simulink subsystem "SelfDefined_Three_Level_NPC_Converter"  (R2024b)
settings: Solver=VariableStepAuto  StartTime=0.0  StopTime=10.0  RelTol=1e-3
libraries: spsIGBTDiodeLib x12, spsDiodeLib x6, simulink x1
settings Model: Creator=XixiLab  LastModifiedBy=XixiLab

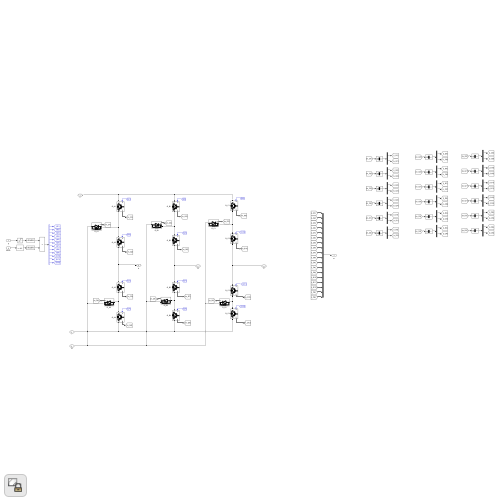
[thumbnail: Simulink's stored preview of the top-level diagram]
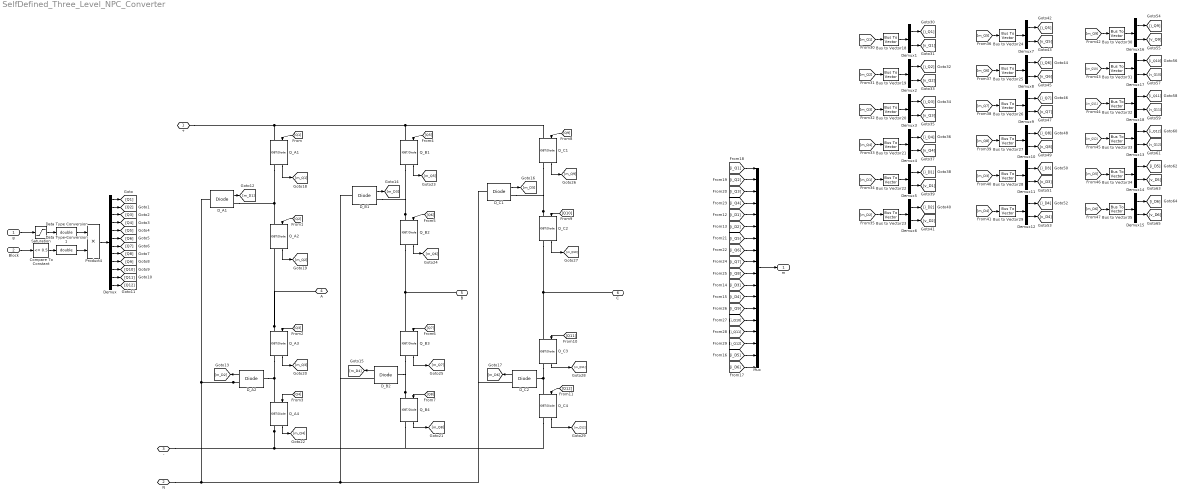
== system SelfDefined_Three_Level_NPC_Converter ==
  g : Inport  PortDimensions=12
  Block : Inport  Port=2  PortDimensions=1
  Bus to Vector{18..35} (18 alike) : BusToVector
  Compare To Constant : simulink/Logic and Bit Operations/Compare To Constant  relop=<=  const=0.5  OutDataTypeStr=boolean
  D_A1 : spsDiodeLib/Diode  Ron=0.001  Lon=0  Vf=0  IC=0  UseSnubber=0  Rs=1e6  Cs=inf  Measurements=on
  D_A2 : spsDiodeLib/Diode  Ron=0.001  Lon=0  Vf=0  IC=0  UseSnubber=0  Rs=1e6  Cs=inf  Measurements=on
  D_B1 : spsDiodeLib/Diode  Ron=0.001  Lon=0  Vf=0  IC=0  UseSnubber=0  Rs=1e6  Cs=inf  Measurements=on
  D_B2 : spsDiodeLib/Diode  Ron=0.001  Lon=0  Vf=0  IC=0  UseSnubber=0  Rs=1e6  Cs=inf  Measurements=on
  D_C1 : spsDiodeLib/Diode  Ron=0.001  Lon=0  Vf=0  IC=0  UseSnubber=0  Rs=1e6  Cs=inf  Measurements=on
  D_C2 : spsDiodeLib/Diode  Ron=0.001  Lon=0  Vf=0  IC=0  UseSnubber=0  Rs=1e6  Cs=inf  Measurements=on
  Data Type Conversion : DataTypeConversion  OutDataTypeStr=double  SaturateOnIntegerOverflow=off  RndMeth=Floor
  Data Type Conversion1 : DataTypeConversion  OutDataTypeStr=double  SaturateOnIntegerOverflow=off  RndMeth=Floor
  Demux : Demux  Outputs=12
  Demux{1..18} (18 alike) : Demux  Outputs=2
  Mux : Mux  Inputs=18
  Product4 : Product
  Q_A{1..4} (4 alike) : spsIGBTDiodeLib/IGBT//Diode  Ron=1e-3  Rs=1e6  Cs=inf  Measurements=on
  Q_B{1..4} (4 alike) : spsIGBTDiodeLib/IGBT//Diode  Ron=1e-3  Rs=1e6  Cs=inf  Measurements=on
  Q_C{1..4} (4 alike) : spsIGBTDiodeLib/IGBT//Diode  Ron=1e-3  Rs=1e6  Cs=inf  Measurements=on
  Saturation : Saturate  UpperLimit=1  LowerLimit=0
  + : PMIOPort  Side=Right
  N : PMIOPort  Port=2  Side=Right
  - : PMIOPort  Port=3  Side=Right
  A : PMIOPort  Port=4  Side=Left
  B : PMIOPort  Port=5  Side=Left
  C : PMIOPort  Port=6  Side=Left
  m : Outport
  wires:
  Demux/10 -> [Q10]
  Data Type Conversion/1 -> Product4/1
  Demux/8 -> [Q8]
  Demux/4 -> [Q4]
  Data Type Conversion1/1 -> Product4/2
  Demux/5 -> [Q5]
  Demux/3 -> [Q3]
  Demux/11 -> [Q11]
  Demux/9 -> [Q9]
  Demux/7 -> [Q7]
  Saturation/1 -> Data Type Conversion/1
  Compare To Constant/1 -> Data Type Conversion1/1
  Demux/6 -> [Q6]
  Product4/1 -> Demux/1
  Demux/12 -> [Q12]
  Demux/2 -> [Q2]
  Demux/1 -> [Q1]
  [Q1] -> Q_A1/1
  [Q2] -> Q_A2/1
  [Q3] -> Q_A3/1
  [Q4] -> Q_A4/1
  [Q6] -> Q_B2/1
  [Q5] -> Q_B1/1
  [Q7] -> Q_B3/1
  [Q8] -> Q_B4/1
  [Q11] -> Q_C3/1
  [Q10] -> Q_C2/1
  [Q12] -> Q_C4/1
  [Q9] -> Q_C1/1
  Block/1 -> Compare To Constant/1
  g/1 -> Saturation/1
  D_A1/1 -> [m_D1]
  D_A2/1 -> [m_D2]
  D_B1/1 -> [m_D3]
  D_B2/1 -> [m_D4]
  D_C1/1 -> [m_D5]
  D_C2/1 -> [m_D6]
  Q_A1/1 -> [m_Q1]
  Q_A2/1 -> [m_Q2]
  Q_A3/1 -> [m_Q3]
  Q_A4/1 -> [m_Q4]
  Q_B1/1 -> [m_Q5]
  Q_B2/1 -> [m_Q6]
  Q_B3/1 -> [m_Q7]
  Q_B4/1 -> [m_Q8]
  Q_C1/1 -> [m_Q9]
  Q_C2/1 -> [m_Q10]
  Q_C3/1 -> [m_Q11]
  Q_C4/1 -> [m_Q12]
  Mux/1 -> m/1
  [i_Q1] -> Mux/1
  [i_Q2] -> Mux/2
  [i_Q3] -> Mux/3
  [i_Q4] -> Mux/4
  [i_D1] -> Mux/5
  [i_D2] -> Mux/6
  [i_Q5] -> Mux/7
  [i_Q6] -> Mux/8
  [i_Q7] -> Mux/9
  [i_Q8] -> Mux/10
  [i_D3] -> Mux/11
  [i_D4] -> Mux/12
  [i_Q9] -> Mux/13
  [i_Q10] -> Mux/14
  [i_Q11] -> Mux/15
  [i_Q12] -> Mux/16
  [i_D5] -> Mux/17
  [i_D6] -> Mux/18
  [m_Q1] -> Bus to Vector18/1
  Bus to Vector18/1 -> Demux1/1
  Demux1/1 -> [i_Q1]
  Demux1/2 -> [v_Q1]
  Demux2/2 -> [v_Q2]
  Bus to Vector19/1 -> Demux2/1
  Demux2/1 -> [i_Q2]
  [m_Q2] -> Bus to Vector19/1
  Demux3/2 -> [v_Q3]
  Bus to Vector20/1 -> Demux3/1
  Demux3/1 -> [i_Q3]
  [m_Q3] -> Bus to Vector20/1
  Demux4/2 -> [v_Q4]
  Bus to Vector21/1 -> Demux4/1
  Demux4/1 -> [i_Q4]
  [m_Q4] -> Bus to Vector21/1
  Demux5/2 -> [v_D1]
  Bus to Vector22/1 -> Demux5/1
  Demux5/1 -> [i_D1]
  [m_D1] -> Bus to Vector22/1
  [m_D2] -> Bus to Vector23/1
  Demux6/1 -> [i_D2]
  Bus to Vector23/1 -> Demux6/1
  Demux6/2 -> [v_D2]
  Demux10/2 -> [v_Q8]
  Bus to Vector27/1 -> Demux10/1
  [m_Q7] -> Bus to Vector26/1
  Demux7/2 -> [v_Q5]
  [m_D3] -> Bus to Vector28/1
  [m_Q6] -> Bus to Vector25/1
  Demux8/2 -> [v_Q6]
  Demux8/1 -> [i_Q6]
  Bus to Vector24/1 -> Demux7/1
  Bus to Vector25/1 -> Demux8/1
  Demux12/2 -> [v_D4]
  Bus to Vector26/1 -> Demux9/1
  Demux11/1 -> [i_D3]
  Demux11/2 -> [v_D3]
  Demux9/1 -> [i_Q7]
  Demux10/1 -> [i_Q8]
  [m_D4] -> Bus to Vector29/1
  Bus to Vector29/1 -> Demux12/1
  Demux12/1 -> [i_D4]
  [m_Q5] -> Bus to Vector24/1
  [m_Q8] -> Bus to Vector27/1
  Demux9/2 -> [v_Q7]
  Demux7/1 -> [i_Q5]
  Bus to Vector28/1 -> Demux11/1
  Bus to Vector34/1 -> Demux14/1
  [m_Q9] -> Bus to Vector30/1
  [m_D6] -> Bus to Vector35/1
  Demux15/1 -> [i_D6]
  [m_Q12] -> Bus to Vector33/1
  Bus to Vector35/1 -> Demux15/1
  Demux18/1 -> [i_Q11]
  Demux14/2 -> [v_D5]
  Demux14/1 -> [i_D5]
  Bus to Vector32/1 -> Demux18/1
  Demux15/2 -> [v_D6]
  Demux18/2 -> [v_Q11]
  Demux13/1 -> [i_Q12]
  Bus to Vector30/1 -> Demux16/1
  Bus to Vector31/1 -> Demux17/1
  Demux17/1 -> [i_Q10]
  Demux16/1 -> [i_Q9]
  Demux17/2 -> [v_Q10]
  [m_Q10] -> Bus to Vector31/1
  [m_D5] -> Bus to Vector34/1
  Demux16/2 -> [v_Q9]
  Bus to Vector33/1 -> Demux13/1
  Demux13/2 -> [v_Q12]
  [m_Q11] -> Bus to Vector32/1
  connections:
  Q_A4/RConn1 -- Q_B4/RConn1 -- Q_C4/RConn1 -- -/RConn1
  Q_A1/LConn1 -- Q_B1/LConn1 -- Q_C1/LConn1 -- +/RConn1
  D_A1/RConn1 -- Q_A2/LConn1 -- Q_A1/RConn1
  D_A2/LConn1 -- Q_A4/LConn1 -- Q_A3/RConn1
  D_A2/RConn1 -- D_B2/RConn1 -- D_B1/LConn1 -- D_C2/RConn1 -- D_C1/LConn1 -- N/RConn1 -- D_A1/LConn1
  Q_B2/LConn1 -- D_B1/RConn1 -- Q_B1/RConn1
  Q_B4/LConn1 -- D_B2/LConn1 -- Q_B3/RConn1
  B/RConn1 -- Q_B3/LConn1 -- Q_B2/RConn1
  D_C2/LConn1 -- Q_C4/LConn1 -- Q_C3/RConn1
  Q_C2/LConn1 -- D_C1/RConn1 -- Q_C1/RConn1
  C/RConn1 -- Q_C3/LConn1 -- Q_C2/RConn1
  Q_A3/LConn1 -- Q_A2/RConn1 -- A/RConn1
